simulink model "FreeAcceleration"  (R2013a)
settings: Solver=ode8  StartTime=0.0  StopTime=0.7  FixedStep=0.0001  RelTol=1e-3
undefined symbols (not defined in the file): B, H, wb, Xm, Xr, Z
settings Model: Creator=Sony  LastModifiedBy=Sony

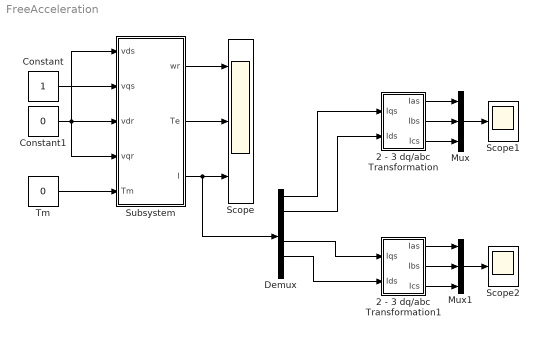
== system FreeAcceleration ==
  2 - 3 dq/abc Transformation : Subsystem
  2 - 3 dq/abc Transformation1 : Subsystem
  Constant : Constant
  Constant1 : Constant  Value=0
  Demux : Demux  Outputs=6
  Mux : Mux  Inputs=3
  Mux1 : Mux  Inputs=3
  Scope : Scope  NumInputPorts=3
      settings: YMin=-2.03e+09~-5~-5  YMax=-1.9975e+09~5~5
  Scope1 : Scope
      settings: YMin=-2.03e+09  YMax=-1.9975e+09
  Scope2 : Scope
      settings: YMin=-2.03e+09  YMax=-1.9975e+09  SaveName=ScopeData2
  Subsystem : Subsystem
  Tm : Constant  Value=0
  wires:
  Constant1/1 -> Subsystem/4(vqr), Subsystem/1(vds), Subsystem/3(vdr)
  Tm/1 -> Subsystem/5(Tm)
  Constant/1 -> Subsystem/2(vqs)
  Subsystem/3(I) -> Demux/1, Scope/3
  Subsystem/2(Te) -> Scope/2
  Subsystem/1(wr) -> Scope/1
  2 - 3 dq/abc Transformation/2(Ibs) -> Mux/2
  2 - 3 dq/abc Transformation/3(Ics) -> Mux/3
  2 - 3 dq/abc Transformation/1(Ias) -> Mux/1
  2 - 3 dq/abc Transformation1/2(Ibs) -> Mux1/2
  2 - 3 dq/abc Transformation1/3(Ics) -> Mux1/3
  2 - 3 dq/abc Transformation1/1(Ias) -> Mux1/1
  Demux/4 -> 2 - 3 dq/abc Transformation1/1(Iqs)
  Demux/5 -> 2 - 3 dq/abc Transformation1/2(Ids)
  Mux/1 -> Scope1/1
  Mux1/1 -> Scope2/1
  Demux/1 -> 2 - 3 dq/abc Transformation/1(Iqs)
  Demux/2 -> 2 - 3 dq/abc Transformation/2(Ids)

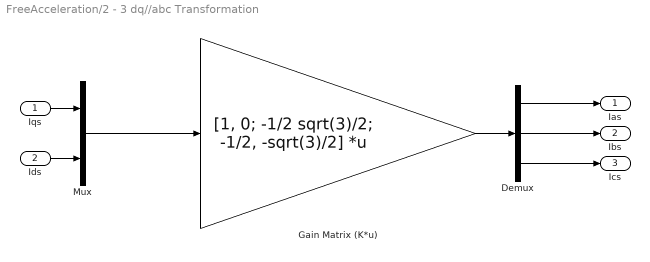
== system FreeAcceleration/2 - 3 dq//abc Transformation ==
  Iqs : Inport
  Ids : Inport  Port=2
  Demux : Demux  Outputs=3
  Gain Matrix (K*u) : Gain  Gain=[1, 0; -1/2 sqrt(3)/2; -1/2, -sqrt(3)/2]  Multiplication=Matrix(K*u)
  Mux : Mux  Inputs=2
  Ias : Outport
  Ibs : Outport  Port=2
  Ics : Outport  Port=3
  wires:
  Mux/1 -> Gain Matrix (K*u)/1
  Gain Matrix (K*u)/1 -> Demux/1
  Demux/2 -> Ibs/1
  Demux/1 -> Ias/1
  Demux/3 -> Ics/1
  Iqs/1 -> Mux/1
  Ids/1 -> Mux/2

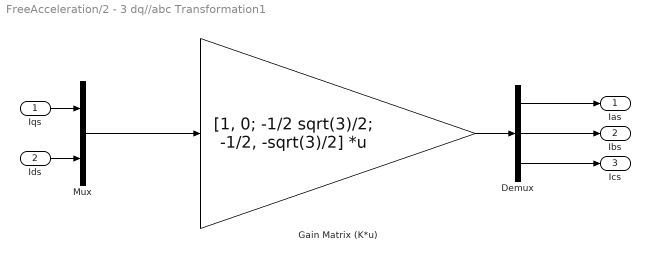
== system FreeAcceleration/2 - 3 dq//abc Transformation1 ==
  Iqs : Inport
  Ids : Inport  Port=2
  Demux : Demux  Outputs=3
  Gain Matrix (K*u) : Gain  Gain=[1, 0; -1/2 sqrt(3)/2; -1/2, -sqrt(3)/2]  Multiplication=Matrix(K*u)
  Mux : Mux  Inputs=2
  Ias : Outport
  Ibs : Outport  Port=2
  Ics : Outport  Port=3
  wires:
  Mux/1 -> Gain Matrix (K*u)/1
  Gain Matrix (K*u)/1 -> Demux/1
  Demux/2 -> Ibs/1
  Demux/1 -> Ias/1
  Demux/3 -> Ics/1
  Iqs/1 -> Mux/1
  Ids/1 -> Mux/2

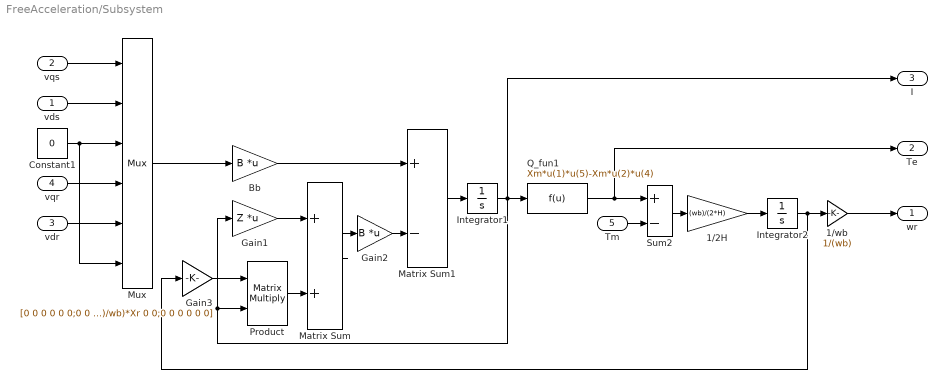
== system FreeAcceleration/Subsystem ==
  vds : Inport
  vqs : Inport  Port=2
  vdr : Inport  Port=3
  vqr : Inport  Port=4
  Tm : Inport  Port=5
  1/2H : Gain  Gain=(wb)/(2*H)
  1/wb : Gain  Gain=1/(wb)
  Bb : Gain  Gain=B  Multiplication=Matrix(K*u)
  Constant1 : Constant  Value=0
  Gain1 : Gain  Gain=Z  Multiplication=Matrix(K*u)
  Gain2 : Gain  Gain=B  Multiplication=Matrix(K*u)
  Gain3 : Gain  Gain=[0 0 0 0 0 0;0 0 0 0 0 0;0 0 0 0 0 0;0 ((-1)/wb)*Xm 0 0 ((-1)/wb)*Xr 0;((1)/wb)*Xm 0 0 ((1)/wb)*Xr 0 0;0 0 0 0 0 0]
  Integrator1 : Integrator  InitialCondition=[0; 0; 0; 0; 0; 0]
  Integrator2 : Integrator
  Matrix Sum : Sum
  Matrix Sum1 : Sum  Inputs=+-
  Mux : Mux  Inputs=6
  Product : Product  Multiplication=Matrix(*)
  Q_fun1 : Fcn  Expr=Xm*u(1)*u(5)-Xm*u(2)*u(4)
  Sum2 : Sum  Inputs=+-  SaturateOnIntegerOverflow=on  InputSameDT=on  OutDataTypeStr=Inherit: Same as first input
  wr : Outport
  Te : Outport  Port=2
  I : Outport  Port=3
  wires:
  Sum2/1 -> 1/2H/1
  vqs/1 -> Mux/1
  Matrix Sum1/1 -> Integrator1/1
  Constant1/1 -> Mux/6, Mux/3
  Tm/1 -> Sum2/2
  Q_fun1/1 -> Te/1, Sum2/1
  vds/1 -> Mux/2
  vdr/1 -> Mux/5
  Mux/1 -> Bb/1
  vqr/1 -> Mux/4
  1/2H/1 -> Integrator2/1
  Gain1/1 -> Matrix Sum/1
  Matrix Sum/1 -> Gain2/1
  Integrator2/1 -> 1/wb/1, Gain3/1
  Gain2/1 -> Matrix Sum1/2
  Product/1 -> Matrix Sum/2
  Integrator1/1 -> I/1, Q_fun1/1, Product/2, Gain1/1
  Bb/1 -> Matrix Sum1/1
  Gain3/1 -> Product/1
  1/wb/1 -> wr/1
